simulink model "test"  (Simulink 7.0)
settings: Solver=ode4  StartTime=0.0  StopTime=10.0  FixedStep=0.01  RelTol=1e-3
libraries: xpclib x3
settings Model: Creator=jporter  LastModifiedBy=jporter  BufferReuse=off
settings OptimizationCC: BlockReduction=off  OptimizeBlockIOStorage=off  BufferReuse=off  ExpressionFolding=off  LocalBlockOutputs=off
settings RTWCC: SystemTargetFile=xpctarget.tlc  TemplateMakefile=xpc_default_tmf  Description=xPC Target  ProcessScript=xpctarget_make_rtw_hook
settings xpcTargetCC: TargetFcnLib=ansi_tfl_table_tmw.mat  GenFloatMathFcnCalls=ANSI_C  CompOptLevelCompliant=off  PortableWordSizes=off  RL32ObjectName=commtest

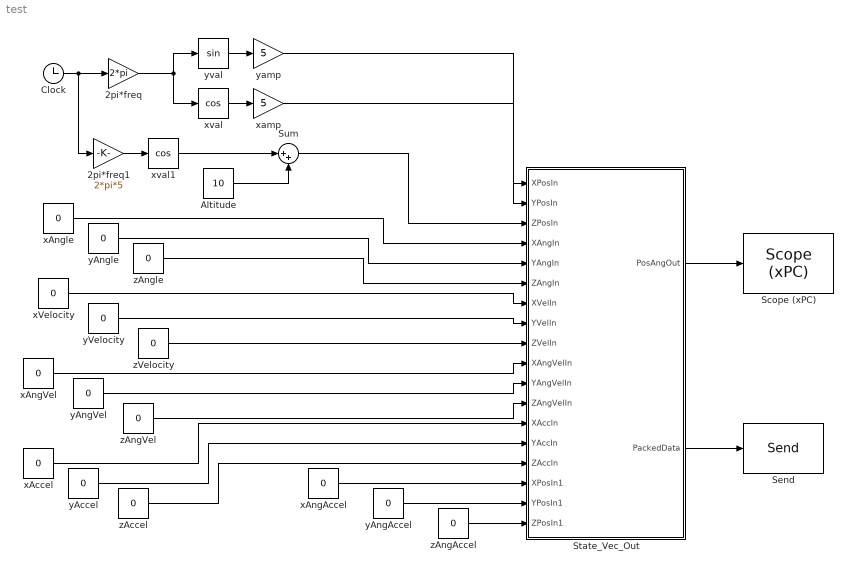
== system test ==
  2pi*freq : Gain  Gain=2*pi  ParameterDataType=sfix(16)  ParameterScaling=2^0  OutDataType=sfix(16)  OutScaling=2^0
  2pi*freq1 : Gain  Gain=2*pi*5  ParameterDataType=sfix(16)  ParameterScaling=2^0  OutDataType=sfix(16)  OutScaling=2^0
  Altitude : Constant  Value=10  OutDataType=sfix(16)  OutScaling=2^0
  Clock : Clock
  "Scope (xPC) " : xpclib/Misc./Scope (xPC)   SystemSampleTime=-1  scopeno=1  scopetype=Target  autostart=on  viewmode=Graphical redraw  formatstr='%15.6f'  grid=on  ylimits=[-12,12]  nosamples=250  noprepostsamples=0  interleave=1  triggermode=FreeRun  triggersignal=1  triggerlevel=0.0  triggerslope=Either  triggerscope=1  triggersample=0  filename=data.dat  mode=Lazy  writesize=512  autorestart=off
  Send : xpclib/UDP/Send  ipAddress=129.59.129.186  ipPort=9877  localPort=-1  sampletime=0.05
  State_Vec_Out : Subsystem
  Sum : Sum  Inputs=|++  OutDataType=sfix(16)  OutScaling=2^0
  xAccel : Constant  Value=0  OutDataType=sfix(16)  OutScaling=2^0
  xAngAccel : Constant  Value=0  OutDataType=sfix(16)  OutScaling=2^0
  xAngVel : Constant  Value=0  OutDataType=sfix(16)  OutScaling=2^0
  xAngle : Constant  Value=0  OutDataType=sfix(16)  OutScaling=2^0
  xVelocity : Constant  Value=0  OutDataType=sfix(16)  OutScaling=2^0
  xamp : Gain  Gain=5  ParameterDataTypeMode=double  ParameterDataType=sfix(16)  ParameterScaling=2^0  OutDataType=sfix(16)  OutScaling=2^0
  xval : Trigonometry  Operator=cos
  xval1 : Trigonometry  Operator=cos
  yAccel : Constant  Value=0  OutDataType=sfix(16)  OutScaling=2^0
  yAngAccel : Constant  Value=0  OutDataType=sfix(16)  OutScaling=2^0
  yAngVel : Constant  Value=0  OutDataType=sfix(16)  OutScaling=2^0
  yAngle : Constant  Value=0  OutDataType=sfix(16)  OutScaling=2^0
  yVelocity : Constant  Value=0  OutDataType=sfix(16)  OutScaling=2^0
  yamp : Gain  Gain=5  ParameterDataTypeMode=double  ParameterDataType=sfix(16)  ParameterScaling=2^0  OutDataType=sfix(16)  OutScaling=2^0
  yval : Trigonometry
  zAccel : Constant  Value=0  OutDataType=sfix(16)  OutScaling=2^0
  zAngAccel : Constant  Value=0  OutDataType=sfix(16)  OutScaling=2^0
  zAngVel : Constant  Value=0  OutDataType=sfix(16)  OutScaling=2^0
  zAngle : Constant  Value=0  OutDataType=sfix(16)  OutScaling=2^0
  zVelocity : Constant  Value=0  OutDataType=sfix(16)  OutScaling=2^0
  wires:
  Clock/1 -> 2pi*freq/1, 2pi*freq1/1
  2pi*freq/1 -> yval/1, xval/1
  yval/1 -> yamp/1
  xval/1 -> xamp/1
  yamp/1 -> State_Vec_Out/1(XPosIn)
  xamp/1 -> State_Vec_Out/2(YPosIn)
  State_Vec_Out/1(PosAngOut) -> "Scope (xPC) "/1
  State_Vec_Out/2(PackedData) -> Send/1
  xAngle/1 -> State_Vec_Out/4(XAngIn)
  yAngle/1 -> State_Vec_Out/5(YAngIn)
  zAngle/1 -> State_Vec_Out/6(ZAngIn)
  xVelocity/1 -> State_Vec_Out/7(XVelIn)
  yVelocity/1 -> State_Vec_Out/8(YVelIn)
  zVelocity/1 -> State_Vec_Out/9(ZVelIn)
  xAngVel/1 -> State_Vec_Out/10(XAngVelIn)
  yAngVel/1 -> State_Vec_Out/11(YAngVelIn)
  zAngVel/1 -> State_Vec_Out/12(ZAngVelIn)
  xAccel/1 -> State_Vec_Out/13(XAccIn)
  yAccel/1 -> State_Vec_Out/14(YAccIn)
  zAccel/1 -> State_Vec_Out/15(ZAccIn)
  xAngAccel/1 -> State_Vec_Out/16(XPosIn1)
  yAngAccel/1 -> State_Vec_Out/17(YPosIn1)
  zAngAccel/1 -> State_Vec_Out/18(ZPosIn1)
  2pi*freq1/1 -> xval1/1
  Sum/1 -> State_Vec_Out/3(ZPosIn)
  xval1/1 -> Sum/1
  Altitude/1 -> Sum/2

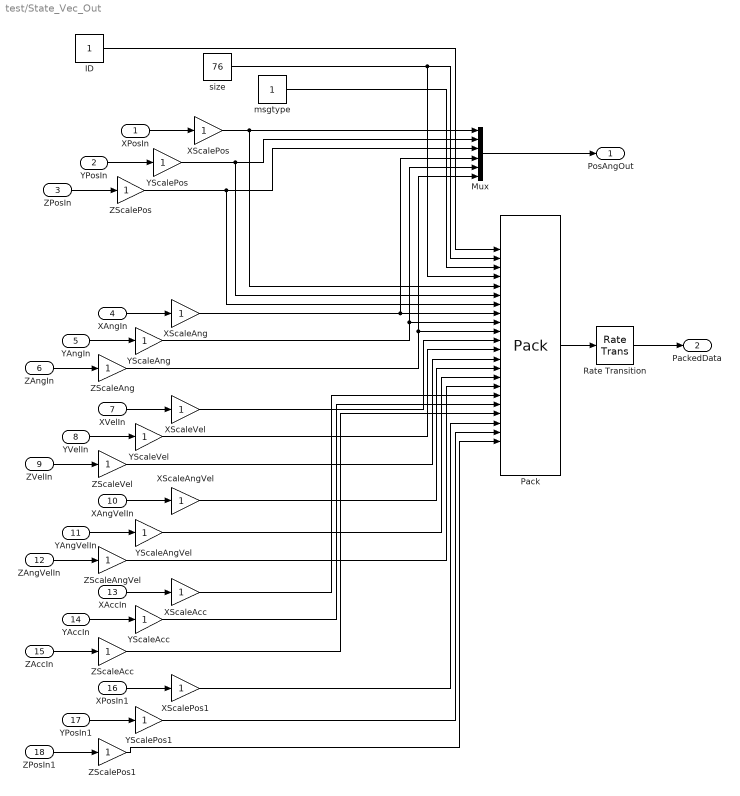
== system test/State_Vec_Out ==
  XPosIn : Inport  OutDataType=sfix(16)  OutScaling=2^0
  YPosIn : Inport  Port=2  OutDataType=sfix(16)  OutScaling=2^0
  ZPosIn : Inport  Port=3  OutDataType=sfix(16)  OutScaling=2^0
  XAngIn : Inport  Port=4  OutDataType=sfix(16)  OutScaling=2^0
  YAngIn : Inport  Port=5  OutDataType=sfix(16)  OutScaling=2^0
  ZAngIn : Inport  Port=6  OutDataType=sfix(16)  OutScaling=2^0
  XVelIn : Inport  Port=7  OutDataType=sfix(16)  OutScaling=2^0
  YVelIn : Inport  Port=8  OutDataType=sfix(16)  OutScaling=2^0
  ZVelIn : Inport  Port=9  OutDataType=sfix(16)  OutScaling=2^0
  XAngVelIn : Inport  Port=10  OutDataType=sfix(16)  OutScaling=2^0
  YAngVelIn : Inport  Port=11  OutDataType=sfix(16)  OutScaling=2^0
  ZAngVelIn : Inport  Port=12  OutDataType=sfix(16)  OutScaling=2^0
  XAccIn : Inport  Port=13  OutDataType=sfix(16)  OutScaling=2^0
  YAccIn : Inport  Port=14  OutDataType=sfix(16)  OutScaling=2^0
  ZAccIn : Inport  Port=15  OutDataType=sfix(16)  OutScaling=2^0
  XPosIn1 : Inport  Port=16  OutDataType=sfix(16)  OutScaling=2^0
  YPosIn1 : Inport  Port=17  OutDataType=sfix(16)  OutScaling=2^0
  ZPosIn1 : Inport  Port=18  OutDataType=sfix(16)  OutScaling=2^0
  ID : Constant  OutDataType=sfix(16)  OutScaling=2^0
  Mux : Mux  Inputs=6
  Pack : xpclib/UDP/Pack  datatypes={'uint32','uint32','uint32','uint32','single','single','single','single','single','single','single','single','single','single','single','single','single','single','single','single','single','single'}  byteAlign=4
  Rate Transition : RateTransition
  XScaleAcc : Gain  ParameterDataType=sfix(16)  ParameterScaling=2^0  OutDataType=sfix(16)  OutScaling=2^0
  XScaleAng : Gain  ParameterDataType=sfix(16)  ParameterScaling=2^0  OutDataType=sfix(16)  OutScaling=2^0
  XScaleAngVel : Gain  ParameterDataType=sfix(16)  ParameterScaling=2^0  OutDataType=sfix(16)  OutScaling=2^0
  XScalePos : Gain  ParameterDataType=sfix(16)  ParameterScaling=2^0  OutDataType=sfix(16)  OutScaling=2^0
  XScalePos1 : Gain  ParameterDataType=sfix(16)  ParameterScaling=2^0  OutDataType=sfix(16)  OutScaling=2^0
  XScaleVel : Gain  ParameterDataType=sfix(16)  ParameterScaling=2^0  OutDataType=sfix(16)  OutScaling=2^0
  YScaleAcc : Gain  ParameterDataType=sfix(16)  ParameterScaling=2^0  OutDataType=sfix(16)  OutScaling=2^0
  YScaleAng : Gain  ParameterDataType=sfix(16)  ParameterScaling=2^0  OutDataType=sfix(16)  OutScaling=2^0
  YScaleAngVel : Gain  ParameterDataType=sfix(16)  ParameterScaling=2^0  OutDataType=sfix(16)  OutScaling=2^0
  YScalePos : Gain  ParameterDataType=sfix(16)  ParameterScaling=2^0  OutDataType=sfix(16)  OutScaling=2^0
  YScalePos1 : Gain  ParameterDataType=sfix(16)  ParameterScaling=2^0  OutDataType=sfix(16)  OutScaling=2^0
  YScaleVel : Gain  ParameterDataType=sfix(16)  ParameterScaling=2^0  OutDataType=sfix(16)  OutScaling=2^0
  ZScaleAcc : Gain  ParameterDataType=sfix(16)  ParameterScaling=2^0  OutDataType=sfix(16)  OutScaling=2^0
  ZScaleAng : Gain  ParameterDataType=sfix(16)  ParameterScaling=2^0  OutDataType=sfix(16)  OutScaling=2^0
  ZScaleAngVel : Gain  ParameterDataType=sfix(16)  ParameterScaling=2^0  OutDataType=sfix(16)  OutScaling=2^0
  ZScalePos : Gain  ParameterDataType=sfix(16)  ParameterScaling=2^0  OutDataType=sfix(16)  OutScaling=2^0
  ZScalePos1 : Gain  ParameterDataType=sfix(16)  ParameterScaling=2^0  OutDataType=sfix(16)  OutScaling=2^0
  ZScaleVel : Gain  ParameterDataType=sfix(16)  ParameterScaling=2^0  OutDataType=sfix(16)  OutScaling=2^0
  msgtype : Constant  OutDataType=sfix(16)  OutScaling=2^0
  size : Constant  Value=76  OutDataType=sfix(16)  OutScaling=2^0
  PosAngOut : Outport  OutDataType=sfix(16)  OutScaling=2^0
  PackedData : Outport  Port=2  OutDataType=sfix(16)  OutScaling=2^0
  wires:
  Pack/1 -> Rate Transition/1
  XScaleAng/1 -> Mux/4, Pack/8
  YScaleAng/1 -> Mux/5, Pack/9
  ZScaleAng/1 -> Mux/6, Pack/10
  ID/1 -> Pack/1
  size/1 -> Pack/2, Pack/4
  msgtype/1 -> Pack/3
  XScaleVel/1 -> Pack/11
  YScaleVel/1 -> Pack/12
  ZScaleVel/1 -> Pack/13
  XScaleAngVel/1 -> Pack/14
  YScaleAngVel/1 -> Pack/15
  ZScaleAngVel/1 -> Pack/16
  XScaleAcc/1 -> Pack/17
  YScaleAcc/1 -> Pack/18
  ZScaleAcc/1 -> Pack/19
  XScalePos1/1 -> Pack/20
  YScalePos1/1 -> Pack/21
  ZScalePos1/1 -> Pack/22
  Mux/1 -> PosAngOut/1
  XPosIn/1 -> XScalePos/1
  YPosIn/1 -> YScalePos/1
  ZPosIn/1 -> ZScalePos/1
  XScalePos/1 -> Mux/1, Pack/5
  YScalePos/1 -> Mux/2, Pack/6
  ZScalePos/1 -> Mux/3, Pack/7
  XAngIn/1 -> XScaleAng/1
  YAngIn/1 -> YScaleAng/1
  ZAngIn/1 -> ZScaleAng/1
  XVelIn/1 -> XScaleVel/1
  YVelIn/1 -> YScaleVel/1
  ZVelIn/1 -> ZScaleVel/1
  XAngVelIn/1 -> XScaleAngVel/1
  YAngVelIn/1 -> YScaleAngVel/1
  ZAngVelIn/1 -> ZScaleAngVel/1
  XAccIn/1 -> XScaleAcc/1
  YAccIn/1 -> YScaleAcc/1
  ZAccIn/1 -> ZScaleAcc/1
  XPosIn1/1 -> XScalePos1/1
  YPosIn1/1 -> YScalePos1/1
  ZPosIn1/1 -> ZScalePos1/1
  Rate Transition/1 -> PackedData/1
